simulink model "ypdqimozuoye"  (Simulink 7.3)
settings: Solver=ode23tb  StartTime=0.0  StopTime=2  RelTol=1e-3
libraries: powerlib x12, powerlib_extras x3
settings Model: Creator=Administrator  LastModifiedBy=Administrator

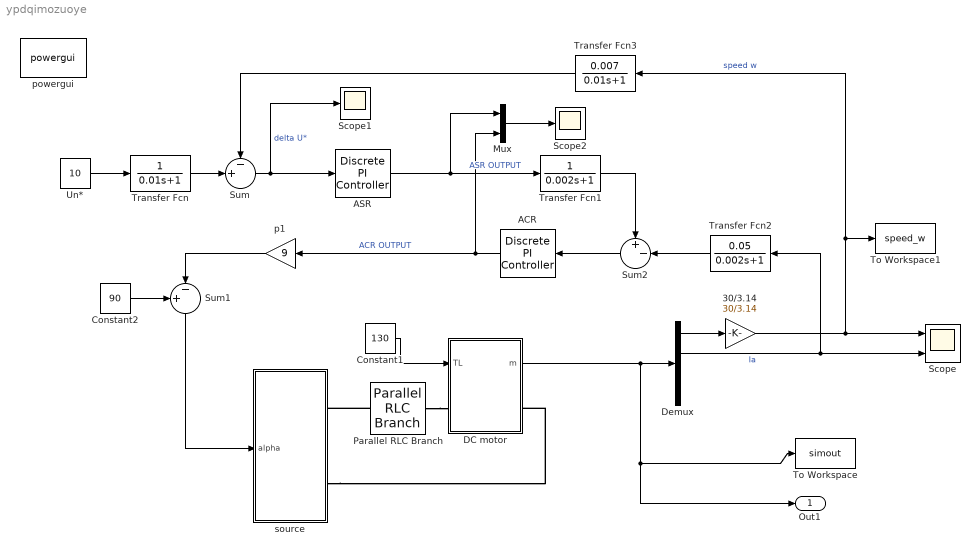
== system ypdqimozuoye ==
  30/3.14 : Gain  Gain=30/3.14  ParameterDataType=fixdt(1, 16)  ParameterScaling=2^0  OutDataType=fixdt(1, 16)  OutScaling=2^0
  ACR : powerlib_extras/Discrete  Control Blocks/Discrete PI Controller  DialogController=POWERSYS.PowerSysDialog  SystemSampleTime=-1  Kp=1.013  Ki=33.77  Par_Limits=[10 0]  Init=0  Ts=50e-6
  ASR : powerlib_extras/Discrete  Control Blocks/Discrete PI Controller  DialogController=POWERSYS.PowerSysDialog  SystemSampleTime=-1  Kp=11.7  Ki=134  Par_Limits=[10 0]  Init=0  Ts=50e-6
  Constant1 : Constant  Value=130  OutDataType=fixdt(1, 16)  OutScaling=2^0
  Constant2 : Constant  Value=90  OutDataType=fixdt(1, 16)  OutScaling=2^0
  DC motor : Subsystem
  Demux : Demux
  Mux : Mux  Inputs=2
  Parallel RLC Branch : powerlib/Elements/Parallel RLC Branch  DialogController=POWERSYS.PowerSysDialog  PhysicalDomain=powersysdomain  SubClassName=unknown  LeftPortType=p1  RightPortType=p1  LConnTagsString=a  RConnTagsString=__new0  BranchType=L  Resistance=1  Inductance=0.015  SetiL0=off  InitialCurrent=0  Capacitance=1e-6  Setx0=off  InitialVoltage=0  Measurements=Branch voltage and current
  Scope : Scope  NumInputPorts=2
      settings: YMin=0~-25  YMax=1500~250
  Scope1 : Scope
      settings: YMin=-0.5  YMax=1
  Scope2 : Scope
      settings: TimeRange=2  YMin=0  YMax=10  SaveName=ScopeData2
  Sum : Sum  Inputs=-+|  OutDataType=fixdt(1, 16)  OutScaling=2^0
  Sum1 : Sum  Inputs=+-|  OutDataType=fixdt(1, 16)  OutScaling=2^0
  Sum2 : Sum  Inputs=+-|  OutDataType=fixdt(1, 16)  OutScaling=2^0
  To Workspace : ToWorkspace  VariableName=simout  SampleTime=-1  SaveFormat=Structure
  To Workspace1 : ToWorkspace  VariableName=speed_w  SampleTime=-1  SaveFormat=Structure With Time
  Transfer Fcn : TransferFcn  Denominator=[0.01 1]
  Transfer Fcn1 : TransferFcn  Denominator=[0.002 1]
  Transfer Fcn2 : TransferFcn  Numerator=0.05  Denominator=[0.002 1]
  Transfer Fcn3 : TransferFcn  Numerator=0.007  Denominator=[0.01 1]
  Un* : Constant  Value=10  OutDataType=fixdt(1, 16)  OutScaling=2^0
  p1 : Gain  Gain=9  ParameterDataType=fixdt(1, 16)  ParameterScaling=2^0  OutDataType=fixdt(1, 16)  OutScaling=2^0
  powergui : powerlib/powergui  Priority=1  SystemSampleTime=-1  SimulationMode=Continuous  SampleTime=50e-6  frequency=60  SPID=off  DisableSnubberDevices=off  DisableRonSwitches=off  DisableVfSwitches=off  SwTol=0  Interpol=off  frequencyindice=0  echomessages=off  HookPort=off  DisplayEquations=off  FunctionMessages=off  EnableUseOfTLC=off  x0status=blocks  RestoreLinks=warning  Frange=[0:2:500]  Ylog=off  Xlog=on  ShowGrid=off  save=off  variable=ZData  ZoomFFT=on  StartTime=0.0  cycles=1  DisplayStyle=1  fundamental=60  FreqAxis=off  MaxFrequency=1000  frequencyindicesteady=1  RmsSteady=1  display=off  Ts=0  methode=off
  source : Subsystem
  Out1 : Outport  OutDataType=fixdt(1, 16)  OutScaling=2^0
  wires:
  DC motor/1(m) -> Demux/1, Out1/1, To Workspace/1
  Demux/2 -> Transfer Fcn2/1, Scope/2  "Ia"
  Demux/1 -> 30/3.14/1
  Un*/1 -> Transfer Fcn/1
  30/3.14/1 -> To Workspace1/1, Transfer Fcn3/1, Scope/1  "speed w"
  Transfer Fcn3/1 -> Sum/1
  Sum/1 -> Scope1/1, ASR/1  "delta U*"
  p1/1 -> Sum1/2
  Constant2/1 -> Sum1/1
  Sum1/1 -> source/1(alpha)
  Constant1/1 -> DC motor/1(TL)
  Transfer Fcn/1 -> Sum/2
  Sum2/1 -> ACR/1
  Transfer Fcn1/1 -> Sum2/1
  Transfer Fcn2/1 -> Sum2/2
  ACR/1 -> p1/1, Mux/2  "ACR OUTPUT"
  Mux/1 -> Scope2/1
  ASR/1 -> Transfer Fcn1/1, Mux/1  "ASR OUTPUT"
  connections:
  Parallel RLC Branch/LConn1 -- source/RConn1
  source/RConn2 -- DC motor/RConn1
  Parallel RLC Branch/RConn1 -- DC motor/LConn1

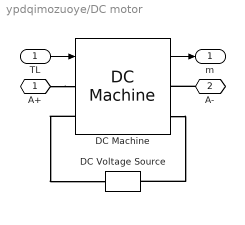
== system ypdqimozuoye/DC motor ==
  TL : Inport
  DC Machine : powerlib/Machines/DC Machine  DialogController=POWERSYS.PowerSysDialog  SystemSampleTime=-1  PresetModel=No  MechanicalLoad=Torque TL  ShowDetailedParameters=on  RLa=[0.2 0.012]  RLf=[240 120]  Laf=1.376  J=0.573  Bm=0  Tf=0  w0=1  Ifinit=0.916666666666667  TsPowergui=0  TsBlock=-1
  DC Voltage Source : powerlib/Electrical Sources/DC Voltage Source  DialogController=POWERSYS.PowerSysDialog  SystemSampleTime=-1  Amplitude=220  Measurements=None
  A+ : PMIOPort  Port=1  Side=Left
  A- : PMIOPort  Port=2  Side=Right
  m : Outport
  wires:
  TL/1 -> DC Machine/1
  DC Machine/1 -> m/1
  connections:
  DC Machine/LConn2 -- DC Voltage Source/RConn1
  DC Machine/RConn2 -- DC Voltage Source/LConn1
  A+/RConn1 -- DC Machine/LConn1
  A-/RConn1 -- DC Machine/RConn1

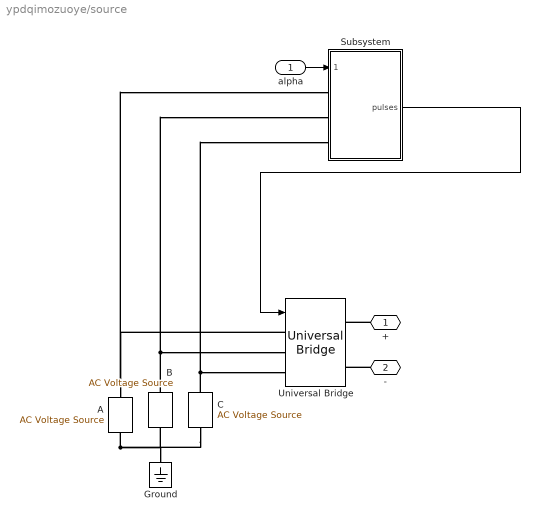
== system ypdqimozuoye/source ==
  alpha : Inport
  A : powerlib/Electrical Sources/AC Voltage Source  DialogController=POWERSYS.PowerSysDialog  SystemSampleTime=-1  Amplitude=220  Phase=0  Frequency=50  SampleTime=0  Measurements=Voltage
  B : powerlib/Electrical Sources/AC Voltage Source  DialogController=POWERSYS.PowerSysDialog  SystemSampleTime=-1  Amplitude=220  Phase=240  Frequency=50  SampleTime=0  Measurements=Voltage
  C : powerlib/Electrical Sources/AC Voltage Source  DialogController=POWERSYS.PowerSysDialog  SystemSampleTime=-1  Amplitude=220  Phase=120  Frequency=50  SampleTime=0  Measurements=Voltage
  Ground : powerlib/Elements/Ground  DialogController=POWERSYS.PowerSysDialog  PhysicalDomain=powersysdomain  SubClassName=unknown  LeftPortType=p1  RightPortType=p1  LConnTagsString=a
  Subsystem : Subsystem
  Universal Bridge : powerlib/Power Electronics/Universal Bridge  DialogController=POWERSYS.PowerSysDialog  SystemSampleTime=-1  Arms=3  SnubberResistance=1e5  SnubberCapacitance=inf  Device=Thyristors  Ron=0.3  Lon=0  ForwardVoltages="[  0  0  ]"  ForwardVoltage=0  GTOparameters=[ 10e-6 , 20e-6 ]  IGBTparameters=[ 1e-6 , 2e-6 ]  Measurements=None  Measurements_2=None  converterType=Rectifier
  + : PMIOPort  Port=1  Side=Right
  - : PMIOPort  Port=2  Side=Right
  wires:
  Subsystem/1(pulses) -> Universal Bridge/1
  alpha/1 -> Subsystem/1(alpha_deg)
  connections:
  A/LConn1 -- C/LConn1 -- B/LConn1 -- Ground/LConn1
  A/RConn1 -- Subsystem/LConn1 -- Universal Bridge/LConn1
  B/RConn1 -- Subsystem/LConn2 -- Universal Bridge/LConn2
  C/RConn1 -- Subsystem/LConn3 -- Universal Bridge/LConn3
  +/RConn1 -- Universal Bridge/RConn1
  -/RConn1 -- Universal Bridge/RConn2

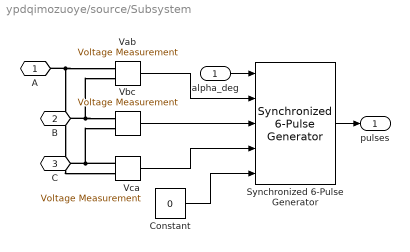
== system ypdqimozuoye/source/Subsystem ==
  alpha_deg : Inport
  Constant : Constant  Value=0  OutDataType=fixdt(1, 16)  OutScaling=2^0
  Synchronized 6-Pulse Generator : powerlib_extras/Control  Blocks/Synchronized 6-Pulse Generator  DialogController=POWERSYS.PowerSysDialog  SystemSampleTime=-1  freq=50  pwidth=10  Double_Pulse=off
  Vab : powerlib/Measurements/Voltage Measurement  DialogController=POWERSYS.PowerSysDialog  SystemSampleTime=-1  PhasorSimulation=off  OutputType=Complex  PSBequivalent=0
  Vbc : powerlib/Measurements/Voltage Measurement  DialogController=POWERSYS.PowerSysDialog  SystemSampleTime=-1  PhasorSimulation=off  OutputType=Complex  PSBequivalent=0
  Vca : powerlib/Measurements/Voltage Measurement  DialogController=POWERSYS.PowerSysDialog  SystemSampleTime=-1  PhasorSimulation=off  OutputType=Complex  PSBequivalent=0
  A : PMIOPort  Port=1  Side=Left
  B : PMIOPort  Port=2  Side=Left
  C : PMIOPort  Port=3  Side=Left
  pulses : Outport
  wires:
  Vab/1 -> Synchronized 6-Pulse Generator/2
  Vbc/1 -> Synchronized 6-Pulse Generator/3
  Vca/1 -> Synchronized 6-Pulse Generator/4
  Constant/1 -> Synchronized 6-Pulse Generator/5
  alpha_deg/1 -> Synchronized 6-Pulse Generator/1
  Synchronized 6-Pulse Generator/1 -> pulses/1
  connections:
  A/RConn1 -- Vca/LConn2 -- Vab/LConn1
  B/RConn1 -- Vbc/LConn1 -- Vab/LConn2
  C/RConn1 -- Vca/LConn1 -- Vbc/LConn2
